simulink model "sampleModel2059_2"  (R2023a)
settings: Solver=VariableStepAuto  StartTime=0.0  StopTime=10.0  RelTol=1e-3
libraries: simulink x4, hdlsllib x2
settings Model: Creator=user1  LastModifiedBy=user1

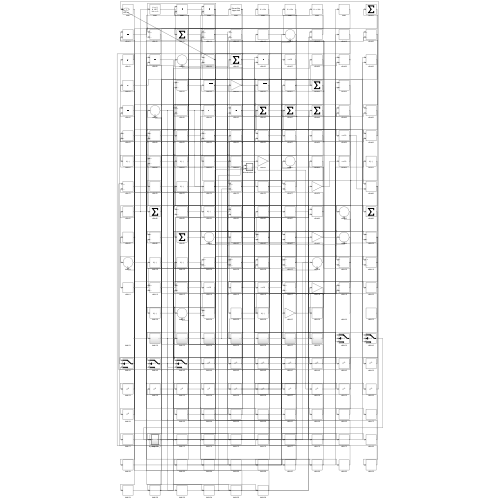
[thumbnail: Simulink's stored preview of the top-level diagram]
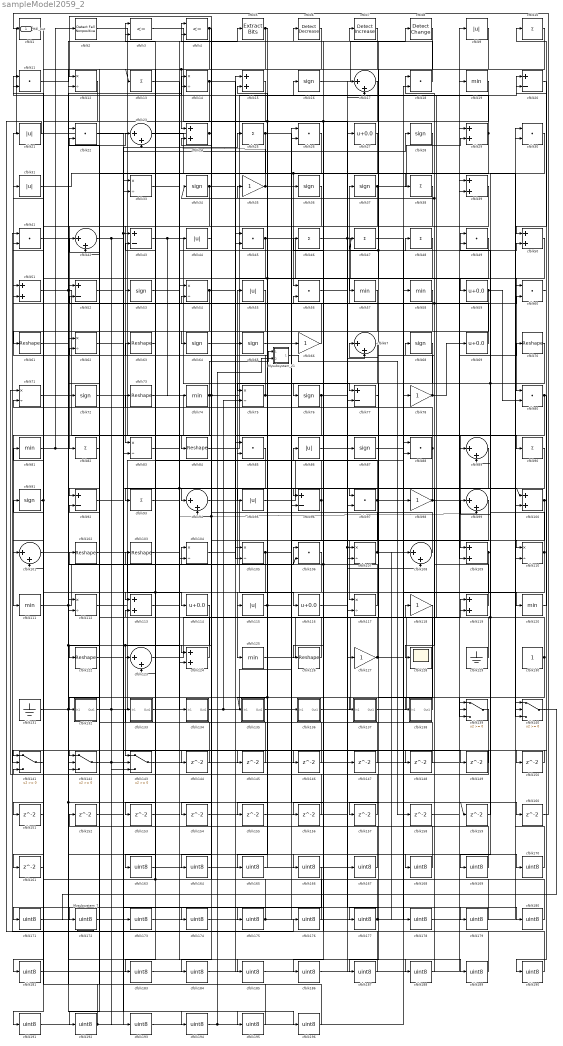
== system sampleModel2059_2 ==
  Mysubsystem_21 : Subsystem  TreatAsAtomicUnit=on  RTWFcnName=Mysubsystem_21
      settings: RTWFcnNameOpts=User specified  RTWFileNameOpts=Use function name
  Mysubsystem_7 : Subsystem  TreatAsAtomicUnit=on  RTWFcnName=Mysubsystem_7
      settings: RTWFcnNameOpts=User specified  RTWFileNameOpts=Use function name
  cfblk1 : hdlsllib/Logic and Bit Operations/Compare To Constant  relop=<=  const=3.0  OutDataTypeStr=uint8
  cfblk{10,13,25,38,46..48,82,90,93} (10 alike) : Sum  Inputs=+  OutDataTypeStr=uint8
  cfblk{15,24,29,39,50..51,100,109,113,119,124} (11 alike) : Sum  OutDataTypeStr=uint8
  cfblk{17,23,42,67,89,94,99,101,108,123} (10 alike) : Sum  Inputs=|++  OutDataTypeStr=uint8
  cfblk{61,63,70,73,84,102..103,122,126} (9 alike) : Reshape
  cfblk{12,14,33,54,62,71,75,83,104..105,107,110,112,117} (14 alike) : Product  Inputs=*/  OutDataTypeStr=uint8  RndMeth=Zero  SaturateOnIntegerOverflow=on
  cfblk{11,18,22,26,30,41,45,49,56,60,80,85,88,97,106} (15 alike) : DotProduct  OutDataTypeStr=uint8
  cfblk{19,57..58,74,81,111,120,125} (8 alike) : MinMax  OutDataTypeStr=uint8
  cfblk{27,59,69,114,116} (5 alike) : Bias  Bias=0.0  SaturateOnIntegerOverflow=off
  cfblk{9,21,31,44,55,86,95,115} (8 alike) : Abs  OutDataTypeStr=uint8  SaturateOnIntegerOverflow=off
  cfblk{35,66,78,98,118,127} (6 alike) : Gain  OutDataTypeStr=uint8
  cfblk128 : Scope
  cfblk129 : Ground
  cfblk130 : Constant  OutDataTypeStr=uint8  SampleTime=-1
  cfblk131 : Ground
  cfblk132 : Subsystem
      settings: LibrarySourceBlock=|
      | hdlsllib/Ports &
      | Subsystems/Subsystem
  cfblk133 : Subsystem
      settings: LibrarySourceBlock=|
      | hdlsllib/Ports &
      | Subsystems/Subsystem
  cfblk134 : Subsystem
      settings: LibrarySourceBlock=|
      | hdlsllib/Ports &
      | Subsystems/Subsystem
  cfblk135 : Subsystem
      settings: LibrarySourceBlock=|
      | hdlsllib/Ports &
      | Subsystems/Subsystem
  cfblk136 : Subsystem
      settings: LibrarySourceBlock=|
      | hdlsllib/Ports &
      | Subsystems/Subsystem
  cfblk137 : Subsystem
      settings: LibrarySourceBlock=|
      | hdlsllib/Ports &
      | Subsystems/Subsystem
  cfblk138 : Subsystem
      settings: LibrarySourceBlock=|
      | hdlsllib/Ports &
      | Subsystems/Subsystem
  cfblk{139..143} (5 alike) : Switch  OutDataTypeStr=uint8  SaturateOnIntegerOverflow=off  InputSameDT=off
  cfblk{144..161} (18 alike) : Delay  SampleTime=1
  cfblk{16,28,34,36..37,53,64..65,68,72,76,87,91} (13 alike) : Signum
  cfblk{163..181,183..196} (33 alike) : DataTypeConversion  OutDataTypeStr=uint8  SaturateOnIntegerOverflow=off  RndMeth=Floor
  cfblk2 : hdlsllib/Logic and Bit Operations/Detect Fall Nonpositive  vinit=0  OutDataTypeStr=uint8
  cfblk{20,43,52,77,92,96} (6 alike) : Sum  Inputs=+-  OutDataTypeStr=uint8
  cfblk3 : RelationalOperator  Operator=<=  OutDataTypeStr=boolean  InputSameDT=off
  cfblk4 : RelationalOperator  Operator=<=  OutDataTypeStr=boolean  InputSameDT=off
  cfblk5 : simulink/Logic and Bit Operations/Extract Bits  bitsToExtract=Upper half  numBits=8  bitIdxRange=[0 7]  outScalingMode=Preserve fixed-point scaling
      settings: LibrarySourceBlock=|
      | hdlsllib/Logic and Bit
      | Operations/Extract Bits
  cfblk6 : simulink/Logic and Bit Operations/Detect Decrease  vinit=0.0  OutDataTypeStr=uint8
      settings: LibrarySourceBlock=|
      | hdlsllib/Logic and Bit
      | Operations/Detect
      | Decrease
  cfblk7 : simulink/Logic and Bit Operations/Detect Increase  vinit=0.0  OutDataTypeStr=uint8
      settings: LibrarySourceBlock=|
      | hdlsllib/Logic and Bit
      | Operations/Detect
      | Increase
  cfblk8 : simulink/Logic and Bit Operations/Detect Change  vinit=0  OutDataTypeStr=uint8
      settings: LibrarySourceBlock=|
      | hdlsllib/Logic and Bit
      | Operations/Detect
      | Change
  Hdl_out : Outport  OutDataTypeStr=uint8
  wires:
  cfblk103/1 -> cfblk175/1
  cfblk4/1 -> cfblk24/1, cfblk13/1, cfblk164/1
  cfblk27/1 -> cfblk56/1, cfblk153/1
  cfblk18/1 -> cfblk12/1
  cfblk137/1(Out1) -> cfblk16/1
  cfblk15/1 -> cfblk111/1
  cfblk106/1 -> cfblk125/1
  cfblk43/1 -> cfblk77/1, cfblk74/1
  cfblk38/1 -> cfblk82/1
  cfblk97/1 -> cfblk102/1, cfblk73/1, cfblk120/1
  cfblk102/1 -> cfblk114/1
  cfblk141/1 -> cfblk81/1
  cfblk51/1 -> cfblk109/1, cfblk23/1
  cfblk135/1(Out1) -> cfblk136/1(In1)
  cfblk84/1 -> cfblk20/1
  cfblk3/1 -> cfblk87/1
  cfblk68/1 -> cfblk177/1
  cfblk111/1 -> cfblk55/1, cfblk60/2
  cfblk98/1 -> cfblk94/1, cfblk70/1
  cfblk36/1 -> cfblk83/1
  cfblk114/1 -> cfblk143/1
  cfblk48/1 -> cfblk132/1(In1), cfblk95/1
  cfblk139/1 -> cfblk71/1
  cfblk131/1 -> cfblk106/1, cfblk168/1
  cfblk142/1 -> cfblk25/1, cfblk193/1
  cfblk70/1 -> cfblk89/1, cfblk156/1
  cfblk105/1 -> cfblk183/1, cfblk191/1, cfblk110/1
  cfblk35/1 -> cfblk23/2, cfblk149/1
  cfblk50/1 -> cfblk80/1
  cfblk75/1 -> cfblk21/1, cfblk139/3
  cfblk138/1(Out1) -> cfblk67/1
  cfblk120/1 -> cfblk20/2
  cfblk101/1 -> cfblk52/1
  cfblk25/1 -> cfblk122/1, cfblk137/1(In1)
  cfblk94/1 -> cfblk116/1
  cfblk72/1 -> cfblk84/1
  cfblk96/1 -> cfblk15/2, cfblk124/1
  cfblk19/1 -> cfblk101/2, cfblk75/1, cfblk76/1
  cfblk64/1 -> cfblk37/1
  cfblk58/1 -> cfblk192/1
  cfblk99/1 -> cfblk117/1
  cfblk132/1(Out1) -> cfblk78/1, cfblk143/3
  cfblk125/1 -> cfblk9/1
  cfblk16/1 -> cfblk8/1
  cfblk2/1 -> cfblk88/2
  cfblk122/1 -> cfblk43/1, cfblk28/1
  cfblk71/1 -> cfblk159/1, cfblk195/1
  cfblk14/1 -> cfblk90/1, cfblk113/1
  cfblk80/1 -> cfblk115/1, cfblk190/1
  cfblk13/1 -> cfblk44/1
  cfblk119/1 -> cfblk34/1, cfblk11/1
  cfblk104/1 -> cfblk48/1
  cfblk127/1 -> cfblk86/1, cfblk50/2
  cfblk63/1 -> cfblk3/1
  cfblk66/1 -> cfblk52/2
  cfblk76/1 -> cfblk117/2, cfblk105/2
  cfblk28/1 -> cfblk126/1
  cfblk42/1 -> cfblk148/1, cfblk173/1
  cfblk123/1 -> cfblk29/1
  cfblk113/1 -> cfblk134/1(In1)
  cfblk115/1 -> cfblk138/1(In1), cfblk65/1
  cfblk69/1 -> cfblk18/1, cfblk6/1
  cfblk129/1 -> cfblk104/1
  cfblk134/1(Out1) -> cfblk66/1, cfblk75/2
  cfblk57/1 -> cfblk64/1
  cfblk112/1 -> cfblk54/1
  cfblk78/1 -> cfblk51/1, cfblk69/1
  cfblk108/1 -> cfblk63/1
  cfblk1/1 -> cfblk141/1
  cfblk55/1 -> cfblk92/1
  cfblk29/1 -> cfblk93/1, cfblk14/2
  cfblk95/1 -> cfblk18/2
  cfblk83/1 -> cfblk100/1, cfblk99/2
  cfblk7/1 -> cfblk53/1
  cfblk100/1 -> cfblk110/2, cfblk150/1
  cfblk136/1(Out1) -> cfblk119/1
  cfblk81/1 -> cfblk123/1, cfblk124/2, cfblk139/2, cfblk2/1
  cfblk45/1 -> cfblk142/2, cfblk140/1
  cfblk53/1 -> cfblk5/1
  cfblk130/1 -> cfblk106/2, cfblk46/1, cfblk99/1, cfblk140/3
  cfblk37/1 -> cfblk29/2, cfblk107/2
  cfblk109/1 -> cfblk135/1(In1), cfblk165/1, cfblk89/2
  cfblk54/1 -> cfblk61/1, cfblk60/1
  cfblk9/1 -> cfblk57/1
  cfblk23/1 -> cfblk100/2
  cfblk77/1 -> cfblk7/1, cfblk47/1
  cfblk6/1 -> cfblk142/3
  cfblk124/1 -> cfblk42/1
  cfblk73/1 -> cfblk107/1, cfblk127/1
  cfblk8/1 -> cfblk101/1
  cfblk88/1 -> cfblk94/2, cfblk174/1, cfblk31/1
  cfblk93/1 -> cfblk104/2
  cfblk61/1 -> cfblk14/1
  cfblk12/1 -> cfblk112/2
  cfblk74/1 -> Mysubsystem_21/1(In1), cfblk54/2, cfblk36/1, cfblk83/2
  cfblk92/1 -> cfblk97/1
  cfblk117/1 -> cfblk24/2
  cfblk46/1 -> cfblk109/2, cfblk59/1
  cfblk133/1(Out1) -> cfblk49/1
  cfblk116/1 -> cfblk108/2
  cfblk10/1 -> cfblk72/1
  cfblk31/1 -> cfblk38/1
  cfblk60/1 -> cfblk10/1
  cfblk62/1 -> cfblk194/1
  cfblk59/1 -> cfblk96/1, cfblk80/2
  cfblk126/1 -> cfblk3/2
  cfblk82/1 -> cfblk42/2
  cfblk34/1 -> cfblk96/2, cfblk143/2
  cfblk90/1 -> cfblk128/1
  cfblk5/1 -> cfblk12/2, cfblk145/1
  cfblk143/1 -> cfblk19/1
  cfblk107/1 -> cfblk71/2, cfblk140/2
  cfblk91/1 -> cfblk41/2, cfblk161/1
  cfblk110/1 -> cfblk49/2, cfblk186/1
  cfblk11/1 -> cfblk4/1
  cfblk20/1 -> cfblk50/1
  cfblk24/1 -> cfblk144/1, Hdl_out/1
  cfblk144/1 -> cfblk92/2
  cfblk145/1 -> cfblk123/2
  cfblk52/1 -> cfblk146/1
  cfblk146/1 -> cfblk105/1
  cfblk147/1 -> cfblk43/2
  cfblk148/1 -> cfblk113/2
  cfblk149/1 -> cfblk142/1
  cfblk150/1 -> cfblk141/2
  cfblk49/1 -> cfblk151/1
  cfblk151/1 -> cfblk51/2
  cfblk44/1 -> cfblk154/1
  cfblk154/1 -> cfblk77/2
  cfblk67/1 -> cfblk155/1
  cfblk155/1 -> cfblk97/2
  cfblk156/1 -> cfblk112/1
  cfblk89/1 -> cfblk157/1
  cfblk157/1 -> cfblk15/1
  cfblk158/1 -> cfblk139/1
  cfblk159/1 -> cfblk119/2
  cfblk65/1 -> cfblk160/1
  cfblk160/1 -> cfblk1/1
  cfblk161/1 -> cfblk141/3
  cfblk85/1 -> cfblk163/1
  cfblk163/1 -> cfblk67/2
  cfblk164/1 -> cfblk85/1
  cfblk165/1 -> cfblk85/2
  cfblk22/1 -> cfblk166/1
  cfblk86/1 -> cfblk167/1
  cfblk167/1 -> cfblk22/1
  cfblk168/1 -> cfblk22/2
  cfblk30/1 -> cfblk169/1
  cfblk169/1 -> cfblk35/1
  cfblk87/1 -> cfblk170/1
  cfblk170/1 -> cfblk30/1
  cfblk166/1 -> cfblk171/1
  cfblk171/1 -> cfblk30/2
  cfblk26/1 -> cfblk172/1
  cfblk172/1 -> cfblk147/1
  cfblk173/1 -> cfblk26/1
  cfblk174/1 -> cfblk26/2
  cfblk175/1 -> cfblk4/2, cfblk88/1
  cfblk21/1 -> cfblk176/1
  cfblk176/1 -> cfblk103/1
  cfblk177/1 -> cfblk11/2, cfblk133/1(In1), cfblk108/1
  cfblk47/1 -> cfblk178/1
  cfblk178/1 -> cfblk68/1
  cfblk152/1 -> cfblk179/1
  cfblk179/1 -> cfblk45/1
  cfblk56/1 -> cfblk180/1
  cfblk180/1 -> cfblk152/1
  cfblk39/1 -> cfblk181/1
  cfblk181/1 -> cfblk45/2
  cfblk183/1 -> cfblk39/2
  cfblk17/1 -> cfblk184/1
  cfblk184/1 -> cfblk27/1
  cfblk153/1 -> cfblk185/1
  cfblk185/1 -> cfblk17/1
  cfblk186/1 -> cfblk17/2
  cfblk118/1 -> cfblk187/1
  cfblk187/1 -> cfblk56/2
  cfblk41/1 -> cfblk188/1
  cfblk188/1 -> cfblk118/1
  cfblk33/1 -> cfblk189/1
  cfblk189/1 -> cfblk41/1
  cfblk190/1 -> cfblk33/1
  cfblk191/1 -> cfblk33/2
  cfblk192/1 -> cfblk91/1, cfblk196/1
  cfblk193/1 -> cfblk58/1
  cfblk194/1 -> Mysubsystem_21/2(In2), cfblk98/1
  cfblk195/1 -> cfblk62/1
  cfblk196/1 -> cfblk62/2
  cfblk140/1 -> Mysubsystem_7/1(In1)
  Mysubsystem_7/1(Out1) -> cfblk39/1
  Mysubsystem_21/1(Out1) -> cfblk158/1

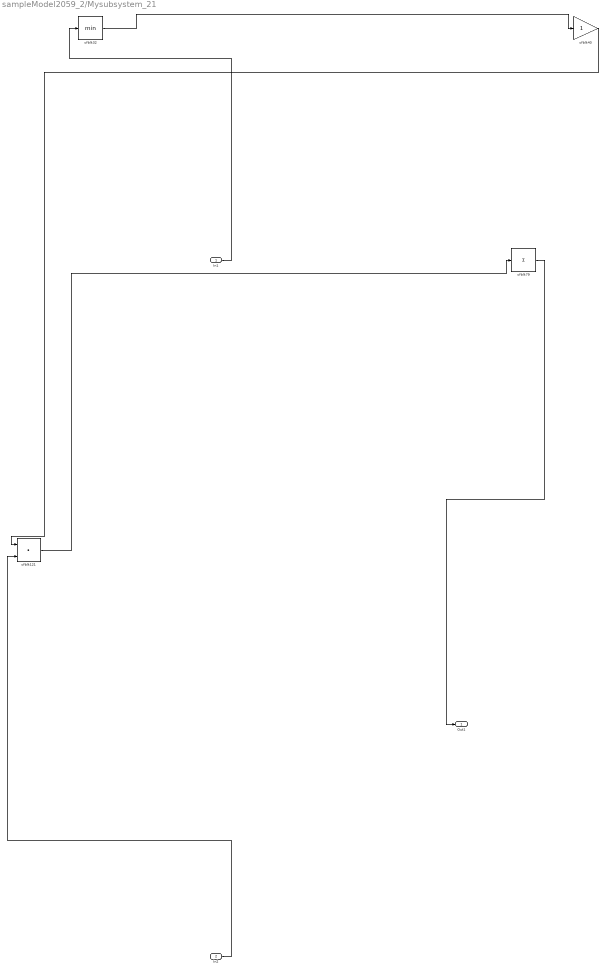
== system sampleModel2059_2/Mysubsystem_21 ==
  In1 : Inport
  In2 : Inport  Port=2
  cfblk121 : DotProduct  OutDataTypeStr=Inherit: Inherit via internal rule
  cfblk32 : MinMax
  cfblk40 : Gain
  cfblk79 : Sum  Inputs=+
  Out1 : Outport
  wires:
  cfblk32/1 -> cfblk40/1
  cfblk40/1 -> cfblk121/1
  In1/1 -> cfblk32/1
  cfblk121/1 -> cfblk79/1
  In2/1 -> cfblk121/2
  cfblk79/1 -> Out1/1

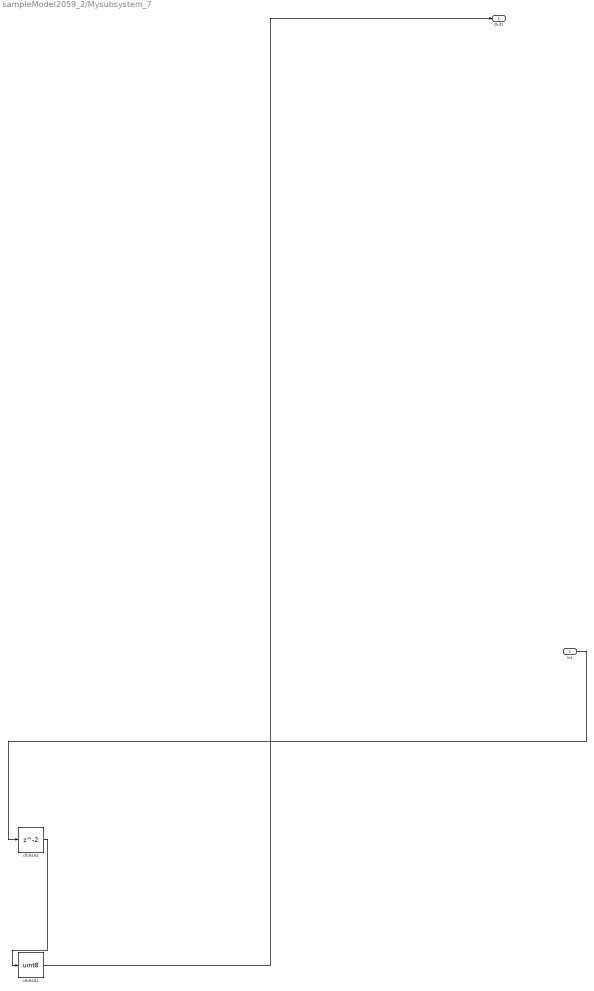
== system sampleModel2059_2/Mysubsystem_7 ==
  In1 : Inport
  cfblk162 : Delay  SampleTime=1
  cfblk182 : DataTypeConversion  OutDataTypeStr=uint8  SaturateOnIntegerOverflow=off  RndMeth=Floor
  Out1 : Outport
  wires:
  cfblk162/1 -> cfblk182/1
  cfblk182/1 -> Out1/1
  In1/1 -> cfblk162/1

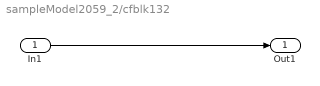
== system sampleModel2059_2/cfblk132 ==
  In1 : Inport
  Out1 : Outport
  wires:
  In1/1 -> Out1/1

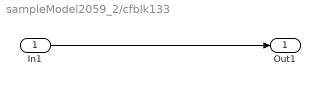
== system sampleModel2059_2/cfblk133 ==
  In1 : Inport
  Out1 : Outport
  wires:
  In1/1 -> Out1/1

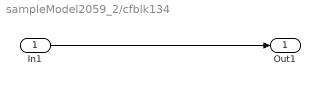
== system sampleModel2059_2/cfblk134 ==
  In1 : Inport
  Out1 : Outport
  wires:
  In1/1 -> Out1/1

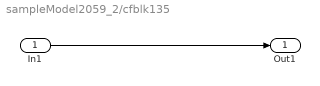
== system sampleModel2059_2/cfblk135 ==
  In1 : Inport
  Out1 : Outport
  wires:
  In1/1 -> Out1/1

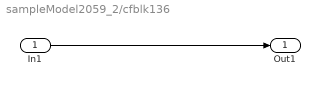
== system sampleModel2059_2/cfblk136 ==
  In1 : Inport
  Out1 : Outport
  wires:
  In1/1 -> Out1/1

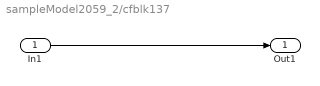
== system sampleModel2059_2/cfblk137 ==
  In1 : Inport
  Out1 : Outport
  wires:
  In1/1 -> Out1/1

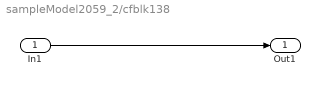
== system sampleModel2059_2/cfblk138 ==
  In1 : Inport
  Out1 : Outport
  wires:
  In1/1 -> Out1/1
